simulink model "sampleModel15"  (R2021b)
settings: Solver=VariableStepAuto  StartTime=0.0  StopTime=10.0  RelTol=1e-3
libraries: simulink x4
settings Model: Creator=user  LastModifiedBy=user

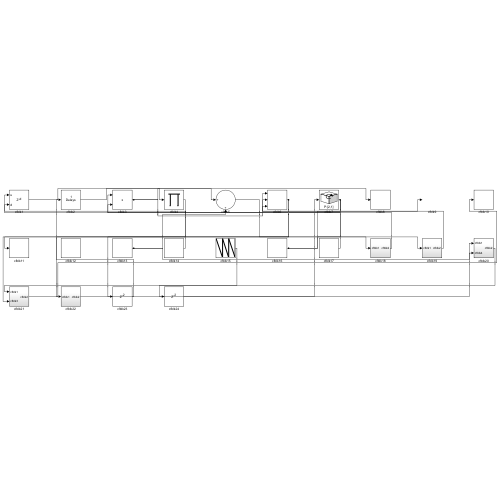
[thumbnail: Simulink's stored preview of the top-level diagram]
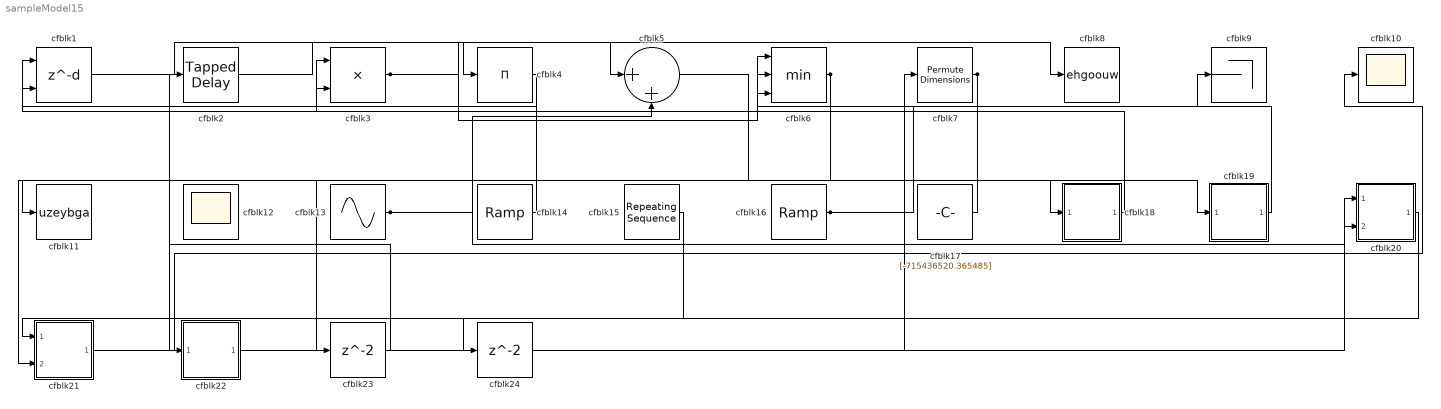
== system sampleModel15 ==
  cfblk1 : Delay  DelayLengthSource=Input port  SampleTime=1
      settings: InputPortMap=u0,p1
  cfblk10 : Scope
  cfblk11 : ToWorkspace  VariableName=uzeybga  SaveFormat=Timeseries  SampleTime=-1
  cfblk12 : Scope
      settings: Floating=on
  cfblk13 : Sin  Amplitude=[343187068.625746]  Bias=[809626460.034724]  SampleTime=0
  cfblk14 : simulink/Sources/Ramp  slope=[1448.326232]  start=[8.617603]  InitialOutput=[4734.867454]
  cfblk15 : simulink/Sources/Repeating Sequence  rep_seq_t=[0 2]  rep_seq_y=[135465756.545948, -623456448.520266]
  cfblk16 : simulink/Sources/Ramp  slope=[-3516.070731]  start=[36.085830]  InitialOutput=[105857.417142]
  cfblk17 : Constant  Value=[-715436520.365485]  SampleTime=1
  cfblk18 : Subsystem
  cfblk19 : Subsystem
  cfblk2 : simulink/Discrete/Tapped Delay  vinit=0.0  samptime=-1  NumDelays=1  DelayOrder=Oldest  includeCurrent=off
  cfblk20 : Subsystem
  cfblk21 : Subsystem
  cfblk22 : Subsystem
  cfblk23 : Delay  SampleTime=1
  cfblk24 : Delay  SampleTime=1
  cfblk3 : Product  Inputs=**
  cfblk4 : Product  Inputs=*
  cfblk5 : Sum  Inputs=|++
  cfblk6 : MinMax  Inputs=3
  cfblk7 : PermuteDimensions
  cfblk8 : ToWorkspace  VariableName=ehgoouw  SaveFormat=Timeseries  SampleTime=-1
  cfblk9 : Terminator
  wires:
  cfblk1/1 -> cfblk4/1
  cfblk4/1 -> cfblk11/1
  cfblk13/1 -> cfblk20/1(cfblk1), cfblk5/2
  cfblk19/1(cfblk2) -> cfblk6/1
  cfblk5/1 -> cfblk19/1(cfblk1)
  cfblk6/1 -> cfblk21/2(cfblk3), cfblk23/1
  cfblk21/1(cfblk2) -> cfblk10/1
  cfblk3/1 -> cfblk8/1, cfblk6/3
  cfblk22/1(cfblk2) -> cfblk20/2(cfblk4)
  cfblk18/1(cfblk2) -> cfblk3/1
  cfblk17/1 -> cfblk3/2
  cfblk15/1 -> cfblk21/1(cfblk1)
  cfblk14/1 -> cfblk1/1
  cfblk16/1 -> cfblk18/1(cfblk1), cfblk9/1
  cfblk2/1 -> cfblk5/1
  cfblk7/1 -> cfblk1/2, cfblk22/1(cfblk1), cfblk6/2
  cfblk23/1 -> cfblk2/1
  cfblk20/1(cfblk2) -> cfblk24/1
  cfblk24/1 -> cfblk7/1

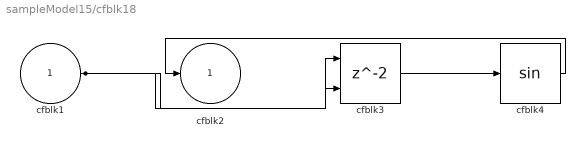
== system sampleModel15/cfblk18 ==
  cfblk1 : Inport
  cfblk3 : Delay  ShowEnablePort=on  SampleTime=1
      settings: InputPortMap=u0,e6
  cfblk4 : Trigonometry
  cfblk2 : Outport
  wires:
  cfblk4/1 -> cfblk2/1
  cfblk3/1 -> cfblk4/1
  cfblk1/1 -> cfblk3/1, cfblk3/2

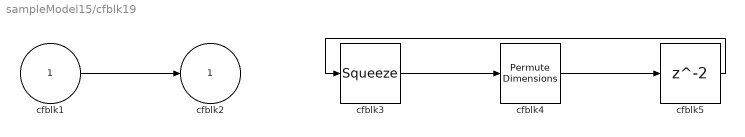
== system sampleModel15/cfblk19 ==
  cfblk1 : Inport
  cfblk3 : Squeeze
  cfblk4 : PermuteDimensions
  cfblk5 : Delay  SampleTime=1
  cfblk2 : Outport
  wires:
  cfblk3/1 -> cfblk4/1
  cfblk1/1 -> cfblk2/1
  cfblk4/1 -> cfblk5/1
  cfblk5/1 -> cfblk3/1

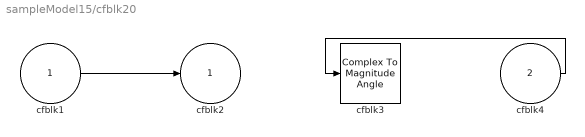
== system sampleModel15/cfblk20 ==
  cfblk1 : Inport
  cfblk4 : Inport  Port=2
  cfblk3 : ComplexToMagnitudeAngle
  cfblk2 : Outport
  wires:
  cfblk4/1 -> cfblk3/1
  cfblk1/1 -> cfblk2/1

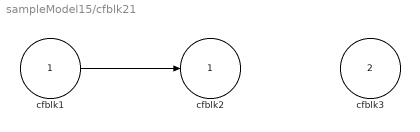
== system sampleModel15/cfblk21 ==
  cfblk1 : Inport
  cfblk3 : Inport  Port=2
  cfblk2 : Outport
  wires:
  cfblk1/1 -> cfblk2/1

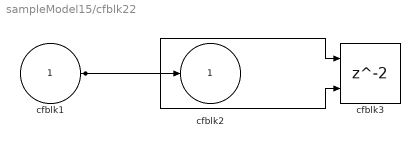
== system sampleModel15/cfblk22 ==
  cfblk1 : Inport
  cfblk3 : Delay  ShowEnablePort=on  SampleTime=1
      settings: InputPortMap=u0,e6
  cfblk2 : Outport
  wires:
  cfblk1/1 -> cfblk2/1, cfblk3/1, cfblk3/2
